simulink model "logical_operators"  (R2022a)
settings: Solver=VariableStepAuto  StartTime=0.0  StopTime=10.0  RelTol=1e-3
settings Model: Creator=Home computer  LastModifiedBy=Home computer

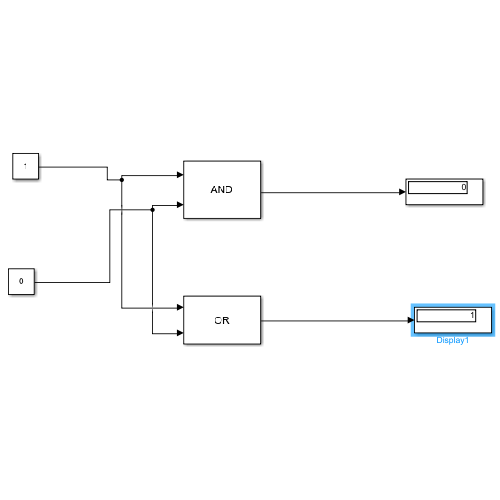
[thumbnail: Simulink's stored preview of the top-level diagram]
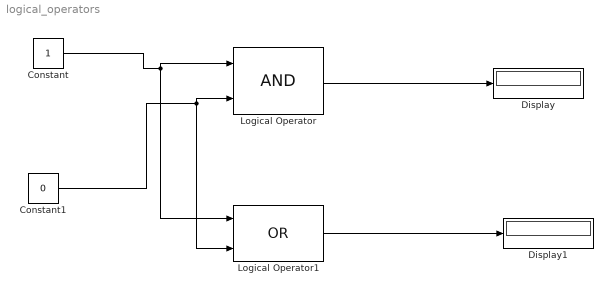
== system logical_operators ==
  Constant : Constant
  Constant1 : Constant  Value=0
  Display : Display
  Display1 : Display
  Logical Operator : Logic  AllPortsSameDT=off  OutDataTypeStr=boolean
  Logical Operator1 : Logic  Operator=OR  AllPortsSameDT=off  OutDataTypeStr=boolean
  wires:
  Constant/1 -> Logical Operator1/1, Logical Operator/1
  Constant1/1 -> Logical Operator1/2, Logical Operator/2
  Logical Operator/1 -> Display/1
  Logical Operator1/1 -> Display1/1
